simulink model "fuzzy"  (Simulink 8.5)
settings: Solver=ode45  StartTime=0.0  StopTime=20  RelTol=1e-3
values from neighbouring files (symbols this model uses):
  A = [-R/L -Kb/L; Km/J -Kf/J]    [main.m]
  B = [1/L; 0]    [main.m]
  b = Kf    (= 0.01)    [main.m]
  C = [0 1]    [main.m]
  gain = 10    [main.m]
  J = J+(rand()-0.5)*J    [main.m]
  K = Kb    (= 0.1)    [main.m]
  K_PP = place(A,B,[p1 p2])    [main.m]
  L = L+(rand()-0.5)*L    [main.m]
  R = R+(rand()-0.5)*R    [main.m]
undefined symbols (not defined in the file): fzy_mdl
settings Model: Creator=dsp520  LastModifiedBy=dsp520
settings DataIOCC: SignalLoggingSaveFormat=Dataset
settings OptimizationCC: ExpressionDepthLimit=128
settings DebuggingCC: UnderspecifiedInitializationDetection=Simplified  MergeDetectMultiDrivingBlocksExec=error  FcnCallInpInsideContextMsg=EnableAllAsError  StateNameClashWarn=none
settings GRTTargetCC: CombineOutputUpdateFcns=on  GRTInterface=off

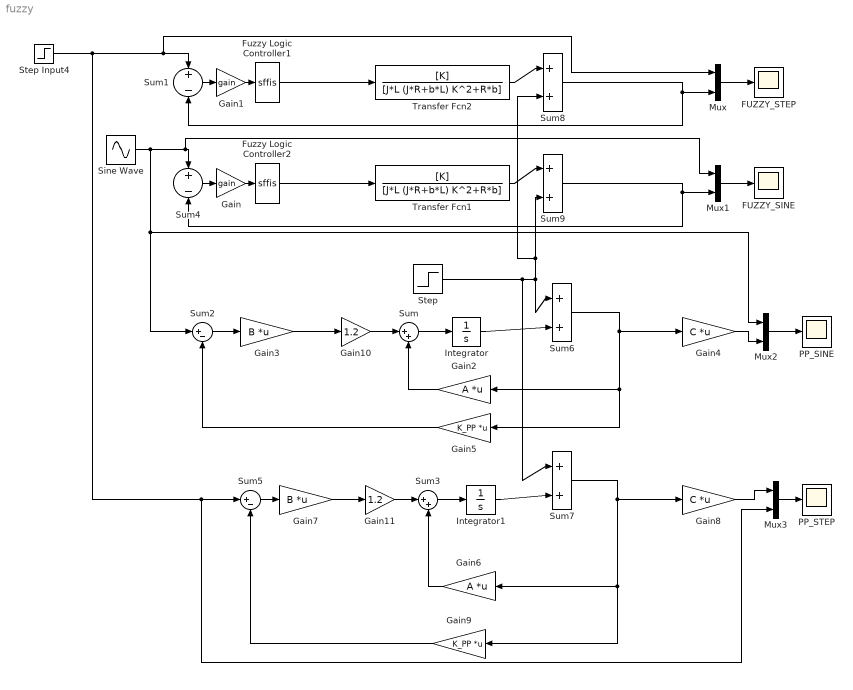
== system fuzzy ==
  "FUZZY_SINE " : Scope
      settings: TimeRange=0.04303388918773621  YMin=1.034906695938528  YMax=1.261470911086717
  FUZZY_STEP : Scope
      settings: TimeRange=20  YMin=0  YMax=2
  Fuzzy Logic Controller1 : S-Function  FunctionName=sffis  Parameters=fismatrix  mask(FIS){fismatrix=fzy_mdl}
      mask prompts: fismatrix "FIS Matrix:"
      mask help: FIS
      mask Help: Fuzzy Inference System
      mask Display: plot(0, -0.3, 6, -0.3, 0, 1.2, 6, 1.2, [0 6], [0 0], [1 2 3],[0 1 0],[2 3 4],[0 1 0],[3 4 5],[0 1 0])
  Fuzzy Logic Controller2 : S-Function  FunctionName=sffis  Parameters=fismatrix  mask(FIS){fismatrix=fzy_mdl}
      mask prompts: fismatrix "FIS Matrix:"
      mask help: FIS
      mask Help: Fuzzy Inference System
      mask Display: plot(0, -0.3, 6, -0.3, 0, 1.2, 6, 1.2, [0 6], [0 0], [1 2 3],[0 1 0],[2 3 4],[0 1 0],[3 4 5],[0 1 0])
  Gain : Gain  Gain=gain
  Gain1 : Gain  Gain=gain
  Gain10 : Gain  Gain=1.2
  Gain11 : Gain  Gain=1.2
  Gain2 : Gain  Gain=A  Multiplication=Matrix(K*u)
  Gain3 : Gain  Gain=B  Multiplication=Matrix(K*u)
  Gain4 : Gain  Gain=C  Multiplication=Matrix(K*u)
  Gain5 : Gain  Gain=K_PP  Multiplication=Matrix(K*u)
  Gain6 : Gain  Gain=A  Multiplication=Matrix(K*u)
  Gain7 : Gain  Gain=B  Multiplication=Matrix(K*u)
  Gain8 : Gain  Gain=C  Multiplication=Matrix(K*u)
  Gain9 : Gain  Gain=K_PP  Multiplication=Matrix(K*u)
  Integrator : Integrator
  Integrator1 : Integrator
  Mux{,1..3} (4 alike) : Mux  Inputs=2
  "PP_SINE " : Scope
      settings: SaveName=ScopeData4
  PP_STEP : Scope
      settings: SaveName=ScopeData2
  Sine Wave : Sin  SampleTime=0
  Step : Step  Time=5  SampleTime=0
  Step Input4 : Step  Time=0
  Sum{,3,6..9} (6 alike) : Sum  Inputs=|++
  Sum1 : Sum  Inputs=+-  SaturateOnIntegerOverflow=on  InputSameDT=on  OutDataTypeStr=Inherit: Same as first input
  Sum2 : Sum  Inputs=|+-
  Sum4 : Sum  Inputs=+-  SaturateOnIntegerOverflow=on  InputSameDT=on  OutDataTypeStr=Inherit: Same as first input
  Sum5 : Sum  Inputs=|+-
  Transfer Fcn1 : TransferFcn  Numerator=[K]  Denominator=[J*L (J*R+b*L) K^2+R*b]
  Transfer Fcn2 : TransferFcn  Numerator=[K]  Denominator=[J*L (J*R+b*L) K^2+R*b]
  wires:
  Fuzzy Logic Controller2/1 -> Transfer Fcn1/1
  Sum4/1 -> Gain/1
  Gain/1 -> Fuzzy Logic Controller2/1
  Fuzzy Logic Controller1/1 -> Transfer Fcn2/1
  Sum1/1 -> Gain1/1
  Gain1/1 -> Fuzzy Logic Controller1/1
  Gain3/1 -> Gain10/1
  Sum2/1 -> Gain3/1
  Integrator/1 -> Sum6/2
  Gain2/1 -> Sum/2
  Gain5/1 -> Sum2/2
  Step Input4/1 -> Mux3/2, Sum5/1, Mux/1, Sum1/1
  Gain7/1 -> Gain11/1
  Sum5/1 -> Gain7/1
  Gain6/1 -> Sum3/2
  Gain9/1 -> Sum5/2
  Step/1 -> Sum8/2, Sum9/2, Sum6/1, Sum7/1
  Sum6/1 -> Gain5/1, Gain2/1, Gain4/1
  Integrator1/1 -> Sum7/2
  Sum7/1 -> Gain9/1, Gain6/1, Gain8/1
  Transfer Fcn2/1 -> Sum8/1
  Sum8/1 -> Mux/2, Sum1/2
  Transfer Fcn1/1 -> Sum9/1
  Mux/1 -> FUZZY_STEP/1
  Mux1/1 -> "FUZZY_SINE "/1
  Sum9/1 -> Mux1/2, Sum4/2
  Mux2/1 -> "PP_SINE "/1
  Sine Wave/1 -> Mux2/1, Sum2/1, Mux1/1, Sum4/1
  Gain4/1 -> Mux2/2
  Mux3/1 -> PP_STEP/1
  Gain8/1 -> Mux3/1
  Sum/1 -> Integrator/1
  Sum3/1 -> Integrator1/1
  Gain11/1 -> Sum3/1
  Gain10/1 -> Sum/1
